simulink model "SimulinkModelDampedTransient"  (R2019a)
settings: Solver=VariableStepAuto  StartTime=0.0  StopTime=10.0  RelTol=1e-3
values from neighbouring files (symbols this model uses):
  alpha = 0    [objective.m]
  beta = 0    [objective.m]
  m1 = 2.294    [MD1.m]    (also in PlotModeShapes.m; animateFlexibleStructure.m; animateFlexibleStructureParFor.m)
  m2 = 1.941    [MD1.m]    (also in PlotModeShapes.m; animateFlexibleStructure.m; animateFlexibleStructureParFor.m)
  m3 = 1.943    [MD1.m]    (also in PlotModeShapes.m; animateFlexibleStructure.m; animateFlexibleStructureParFor.m)
  m4 = 2.732    [MD1.m]    (also in PlotModeShapes.m; animateFlexibleStructure.m; animateFlexibleStructureParFor.m)
  m5 = 0.774    [MD1.m]    (also in PlotModeShapes.m; animateFlexibleStructure.m; animateFlexibleStructureParFor.m)
  m6 = 0.774    [MD1.m]    (also in PlotModeShapes.m; animateFlexibleStructure.m; animateFlexibleStructureParFor.m)
undefined symbols (not defined in the file or in its folder): k1, k2, k3, k4, k5, k6, sf
settings Model: Creator=JacobOesterby  LastModifiedBy=JacobOesterby

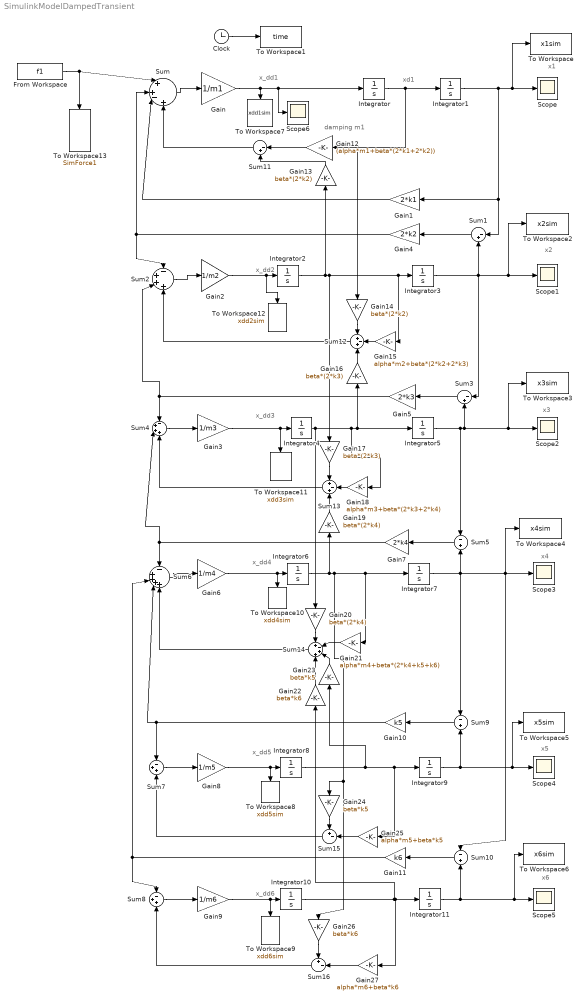
== system SimulinkModelDampedTransient ==
  note: x3
  note: x5
  note: x_dd4
  note: x2
  note: x_dd2
  note: xd1
  note: x6
  note: damping m1
  note: x_dd1
  note: x_dd5
  note: x_dd6
  note: x1
  note: x4
  note: x_dd3
  Clock : Clock
  From Workspace : FromWorkspace  VariableName=f1  OutDataTypeStr=double  SampleTime=sf  Interpolate=off  OutputAfterFinalValue=Setting to zero
  Gain : Gain  Gain=1/m1
  Gain1 : Gain  Gain=2*k1
  Gain10 : Gain  Gain=k5
  Gain11 : Gain  Gain=k6
  Gain12 : Gain  Gain=(alpha*m1+beta*(2*k1+2*k2))
  Gain13 : Gain  Gain=beta*(2*k2)
  Gain14 : Gain  Gain=beta*(2*k2)
  Gain15 : Gain  Gain=alpha*m2+beta*(2*k2+2*k3)
  Gain16 : Gain  Gain=beta*(2*k3)
  Gain17 : Gain  Gain=beta*(2*k3)
  Gain18 : Gain  Gain=alpha*m3+beta*(2*k3+2*k4)
  Gain19 : Gain  Gain=beta*(2*k4)
  Gain2 : Gain  Gain=1/m2
  Gain20 : Gain  Gain=beta*(2*k4)
  Gain21 : Gain  Gain=alpha*m4+beta*(2*k4+k5+k6)
  Gain22 : Gain  Gain=beta*k6
  Gain23 : Gain  Gain=beta*k5
  Gain24 : Gain  Gain=beta*k5
  Gain25 : Gain  Gain=alpha*m5+beta*k5
  Gain26 : Gain  Gain=beta*k6
  Gain27 : Gain  Gain=alpha*m6+beta*k6
  Gain3 : Gain  Gain=1/m3
  Gain4 : Gain  Gain=2*k2
  Gain5 : Gain  Gain=2*k3
  Gain6 : Gain  Gain=1/m4
  Gain7 : Gain  Gain=2*k4
  Gain8 : Gain  Gain=1/m5
  Gain9 : Gain  Gain=1/m6
  Integrator{,1..11} (12 alike) : Integrator
  Scope{,1..6} (7 alike) : Scope
  Sum : Sum  Inputs=|+|+-|+
  Sum1 : Sum  Inputs=|-+
  Sum10 : Sum  Inputs=-+
  Sum11 : Sum  Inputs=|-+
  Sum12 : Sum  Inputs=+-+
  Sum13 : Sum  Inputs=+-+
  Sum14 : Sum  Inputs=+-++
  Sum15 : Sum  Inputs=+-|
  Sum16 : Sum  Inputs=+-|
  Sum2 : Sum  Inputs=-+++
  Sum3 : Sum  Inputs=|-+
  Sum4 : Sum  Inputs=-+++
  Sum5 : Sum  Inputs=-+
  Sum6 : Sum  Inputs=-|++++
  Sum7 : Sum  Inputs=-++
  Sum8 : Sum  Inputs=-++
  Sum9 : Sum  Inputs=-+
  To Workspace : ToWorkspace  VariableName=x1sim  SampleTime=sf
  To Workspace1 : ToWorkspace  VariableName=time  SampleTime=sf
  To Workspace10 : ToWorkspace  VariableName=xdd4sim  SampleTime=sf
  To Workspace11 : ToWorkspace  VariableName=xdd3sim  SampleTime=sf
  To Workspace12 : ToWorkspace  VariableName=xdd2sim  SampleTime=sf
  To Workspace13 : ToWorkspace  VariableName=SimForce1  SampleTime=sf
  To Workspace2 : ToWorkspace  VariableName=x2sim  SampleTime=sf
  To Workspace3 : ToWorkspace  VariableName=x3sim  SampleTime=sf
  To Workspace4 : ToWorkspace  VariableName=x4sim  SampleTime=sf
  To Workspace5 : ToWorkspace  VariableName=x5sim  SampleTime=sf
  To Workspace6 : ToWorkspace  VariableName=x6sim  SampleTime=sf
  To Workspace7 : ToWorkspace  VariableName=xdd1sim  SampleTime=sf
  To Workspace8 : ToWorkspace  VariableName=xdd5sim  SampleTime=sf
  To Workspace9 : ToWorkspace  VariableName=xdd6sim  SampleTime=sf
  wires:
  Integrator10/1 -> Gain27/1, Integrator11/1, Gain22/1
  Sum10/1 -> Gain11/1
  Sum3/1 -> Gain5/1
  Gain5/1 -> Sum4/1, Sum2/3
  Sum6/1 -> Gain6/1
  Sum7/1 -> Gain8/1
  Integrator1/1 -> To Workspace/1, Scope/1, Gain1/1, Sum1/1
  Gain10/1 -> Sum6/4, Sum7/1
  Gain16/1 -> Sum12/3
  Gain/1 -> Scope6/1, Integrator/1, To Workspace7/1
  Gain3/1 -> To Workspace11/1, Integrator4/1
  Integrator3/1 -> Sum1/2, To Workspace2/1, Scope1/1, Sum3/1
  Clock/1 -> To Workspace1/1
  Integrator9/1 -> To Workspace5/1, Scope4/1, Sum9/2
  Sum8/1 -> Gain9/1
  Gain11/1 -> Sum6/3, Sum8/1
  Integrator8/1 -> Gain25/1, Integrator9/1, Gain23/1
  Sum16/1 -> Sum8/3
  Sum1/1 -> Gain4/1
  Integrator7/1 -> Sum9/1, To Workspace4/1, Scope3/1, Sum10/1, Sum5/2
  Gain7/1 -> Sum4/3, Sum6/1
  Integrator5/1 -> To Workspace3/1, Scope2/1, Sum3/2, Sum5/1
  Integrator2/1 -> Gain15/1, Integrator3/1, Gain17/1, Gain13/1
  Sum5/1 -> Gain7/1
  Gain12/1 -> Sum11/1
  Gain8/1 -> To Workspace8/1, Integrator8/1
  Gain15/1 -> Sum12/2
  Integrator4/1 -> Gain18/1, Integrator5/1, Gain16/1, Gain20/1
  Sum/1 -> Gain/1
  Sum12/1 -> Sum2/4
  Gain20/1 -> Sum14/1
  Integrator6/1 -> Gain19/1, Integrator7/1, Gain21/1, Gain26/1, Gain24/1
  Gain19/1 -> Sum13/3
  Sum9/1 -> Gain10/1
  Integrator/1 -> Gain12/1, Gain14/1, Integrator1/1
  Sum13/1 -> Sum4/4
  Gain17/1 -> Sum13/1
  Gain9/1 -> To Workspace9/1, Integrator10/1
  Gain23/1 -> Sum14/3
  Sum11/1 -> Sum/4
  Gain4/1 -> Sum2/1, Sum/2
  Sum2/1 -> Gain2/1
  Gain22/1 -> Sum14/4
  Sum14/1 -> Sum6/5
  Gain18/1 -> Sum13/2
  Gain24/1 -> Sum15/1
  Gain14/1 -> Sum12/1
  Gain25/1 -> Sum15/2
  Sum4/1 -> Gain3/1
  Sum15/1 -> Sum7/3
  Gain26/1 -> Sum16/1
  Integrator11/1 -> To Workspace6/1, Scope5/1, Sum10/2
  Gain27/1 -> Sum16/2
  Gain1/1 -> Sum/3
  From Workspace/1 -> To Workspace13/1, Sum/1
  Gain21/1 -> Sum14/2
  Gain6/1 -> To Workspace10/1, Integrator6/1
  Gain13/1 -> Sum11/2
  Gain2/1 -> To Workspace12/1, Integrator2/1
